simulink model "week_1_springmass_systemmodel"  (R2020b)
settings: Solver=VariableStepAuto  StartTime=0.0  StopTime=10.0  RelTol=1e-3
undefined symbols (not defined in the file): b, k, Kd, Ki, Kp, m, Step_value
settings Model: Creator=anime  LastModifiedBy=anime

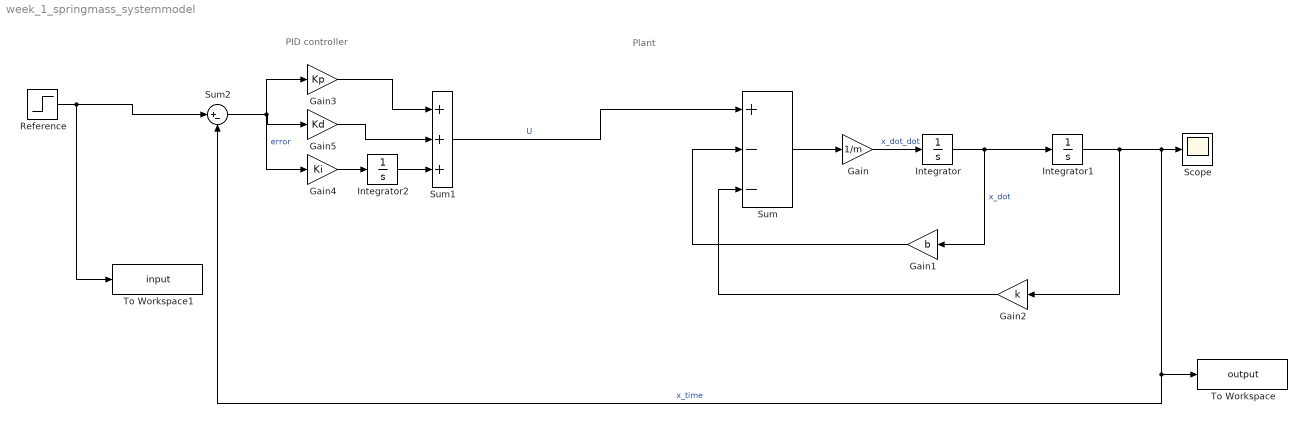
== system week_1_springmass_systemmodel ==
  note: Plant
  note: PID controller
  Gain : Gain  Gain=1/m
  Gain1 : Gain  Gain=b
  Gain2 : Gain  Gain=k
  Gain3 : Gain  Gain=Kp
  Gain4 : Gain  Gain=Ki
  Gain5 : Gain  Gain=Kd
  Integrator : Integrator
  Integrator1 : Integrator
  Integrator2 : Integrator
  Reference : Step  After=Step_value  SampleTime=0
  Scope : Scope
  Sum : Sum  Inputs=|+--
  Sum1 : Sum  Inputs=+++
  Sum2 : Sum  Inputs=|+-
  To Workspace : ToWorkspace  VariableName=output  SaveFormat=Timeseries  SampleTime=-1
  To Workspace1 : ToWorkspace  VariableName=input  SaveFormat=Timeseries  SampleTime=-1
  wires:
  Sum/1 -> Gain/1
  Gain/1 -> Integrator/1  "x_dot_dot"
  Integrator/1 -> Gain1/1, Integrator1/1  "x_dot"
  Integrator1/1 -> To Workspace/1, Sum2/2, Scope/1, Gain2/1  "x_time"
  Gain1/1 -> Sum/2
  Gain2/1 -> Sum/3
  Gain3/1 -> Sum1/1
  Gain4/1 -> Integrator2/1
  Integrator2/1 -> Sum1/3
  Gain5/1 -> Sum1/2
  Sum1/1 -> Sum/1  "U"
  Reference/1 -> To Workspace1/1, Sum2/1
  Sum2/1 -> Gain4/1, Gain3/1, Gain5/1  "error"
